simulink model "serial_i2c_sensors_MPU9250"  (R2015a)
settings: Solver=FixedStepDiscrete  SolverMode=SingleTasking  StartTime=0.0  StopTime=10.0  FixedStep=1e-3  RelTol=1e-3
libraries: mbed_lib x4, mbed_i2c_sensors x3
settings Model: CovSFcnEnable=off  Creator=Sven Lack  LastModifiedBy=oh
settings OptimizationCC: OptimizeModelRefInitCode=on  LifeSpan=1
settings DebuggingCC: SolverPrmCheckMsg=warning
settings HardwareCC: ProdLargestAtomicInteger=Long  ProdLargestAtomicFloat=Double  ProdEndianess=LittleEndian  ProdHWDeviceType=ARM Compatible->ARM Cortex
settings RTWCC: SystemTargetFile=mbed.tlc  TemplateMakefile=mbed.tmf  Description=Mbed Target (Embedded Target)  TargetLang=C++
settings CodeAppCC: IgnoreCustomStorageClasses=off
settings STFCustomTargetCC: CombineOutputUpdateFcns=on  SupportContinuousTime=off  SupportVariableSizeSignals=off  SystemTargetFile=mbed.tlc
settings ERTTargetCC: SupportContinuousTime=off  SupportVariableSizeSignals=off  ERTCustomFileTemplate=mbed_file_process.tlc

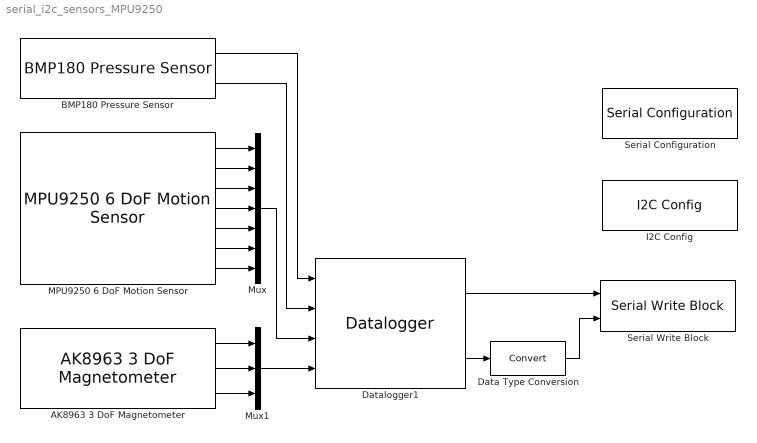
== system serial_i2c_sensors_MPU9250 ==
  AK8963 3 DoF Magnetometer : mbed_i2c_sensors/AK8963 3 DoF Magnetometer  i2cbus=1  SubAddress=0x18  SampleTime=-1
  BMP180 Pressure Sensor : mbed_i2c_sensors/BMP180 Pressure Sensor  i2cbus=1  SampleTime=-1
  Data Type Conversion : DataTypeConversion
  Datalogger1 : mbed_lib/Utilities/Datalogger  TypeInputPorts={ 'int32' 1 'double' 1 'double' 7 'double' 3 }  TypeOfInputs={'1*int32' '1*double' '7*double' '3*double'}  BufferSize=1000  errEn=off  SampleTime=0.01
  I2C Config : mbed_lib/Serial/I2C/I2C Config  Priority=0  I2cPort=1  SParameter6=100000  SParameter2=B  SParameter3=9  SParameter4=B  SParameter5=8
  MPU9250 6 DoF Motion Sensor : mbed_i2c_sensors/MPU9250 6 DoF Motion Sensor  i2cbus=1  SubAddress=0xD0  SampleTime=0.01
  Mux : Mux  Inputs=7
  Mux1 : Mux  Inputs=3
  Serial Configuration : mbed_lib/Serial/UART/Serial Configuration  SerialPort=1  TXPort=A  TXPin=2  RXPort=A  RXPin=3  BaudRate=9600
  Serial Write Block : mbed_lib/Serial/UART/Serial Write Block  SerialPort=1  numData=on  SampleTime=-1
  wires:
  Datalogger1/1 -> Serial Write Block/1
  BMP180 Pressure Sensor/2 -> Datalogger1/2
  BMP180 Pressure Sensor/1 -> Datalogger1/1
  Datalogger1/2 -> Data Type Conversion/1
  Data Type Conversion/1 -> Serial Write Block/2
  Mux/1 -> Datalogger1/3
  MPU9250 6 DoF Motion Sensor/2 -> Mux/2
  MPU9250 6 DoF Motion Sensor/1 -> Mux/1
  MPU9250 6 DoF Motion Sensor/7 -> Mux/7
  MPU9250 6 DoF Motion Sensor/4 -> Mux/4
  MPU9250 6 DoF Motion Sensor/6 -> Mux/6
  MPU9250 6 DoF Motion Sensor/3 -> Mux/3
  MPU9250 6 DoF Motion Sensor/5 -> Mux/5
  AK8963 3 DoF Magnetometer/1 -> Mux1/1
  AK8963 3 DoF Magnetometer/2 -> Mux1/2
  Mux1/1 -> Datalogger1/4
  AK8963 3 DoF Magnetometer/3 -> Mux1/3
